simulink model "fivezonevav"  (R2020a)
settings: Solver=FixedStepAuto  StartTime=0  StopTime=2*24*3600  FixedStep=0.1  RelTol=1e-3
PostLoadFcn:
  | if any(exist('dsrtsu_mdlpostloadfcn', 'file') ~= 0), dsrtsu_mdlpostloadfcn('Execute', bdroot); end
InitFcn:
  | , if any(exist('rtifpga_mdlclblib', 'file') ~= 0), rtifpga_mdlclblib('Init', bdroot); end,
  | , if any(exist('dsmpb_private', 'file') ~= 0), dsmpb_private('dsmpb_mdlclblib', 'Init', bdroot); end,
undefined symbols (not defined in the file): dspaceexample_f_dy9753g2x2M
PreSaveFcn:
  | , if any(exist('dsmpb_private', 'file') ~= 0), dsmpb_private('dsmpb_mdlclblib', 'PreSave', bdroot); end,
CloseFcn:
  | , if any(exist('dsmpb_private', 'file') ~= 0), dsmpb_private('dsmpb_mdlclblib', 'Close', bdroot); end,
settings Model: RTICANMMDATA=struct('GeneralSetupData',struct('modelroot','D:\github\dspace-modelica-example\simulink\fivezone','generalsettings',struct('filesettings',struct('destfolder',struct('Name','RTICANMM_FILES','Check',1),'buildfolder',struct('Name','.','Check',1),'AbsDestfolder',struct('Name','D:\github\dspace-modelica-example\simulink\fivezone\RTICANMM_FILES'),'AbsBuildfolder',struct('Name','D:\github\dspace-modelica-example\simulink\fivezone'))),'options',struct('addpaths',1,'rmpaths',1,'addtrcexclusion',true,'cannavigator',struct('checkmonitoring',0),'show_usrtrc',0,'use_usrtrc',0),'advanced',struct('options',ones(1,100)),'MPSetup',{{}},'RTI',struct('Type','DSRT','Ver','4.3','Date','02-May-2020'),'modelname','fivezonevav','block','fivezonevav'))  DSRTSU_INTERNAL_RTIFPGA=160  DSMPB_ID_DATA={'100',struct('BlockId','6dd11bb4-ebec-4f08-8ba6-7ddbcbec7d3b','SignalIds',{{'2fb2bb90-4ec6-48ad-8f81-f1d196760c71'}}),'101',struct('BlockId','2ef807c6-571a-44f3-9a64-946af00fb830','SignalIds',{{'b929fcdd-48af-480b-af6b-b2c3ef490cf9'}}),'102',struct('BlockId','fcb8ffc9-48d0-43e3-97e6-63db34e8a87a','SignalIds',{{'7405cf0b-34b8-4d18-b681-bf257a32f1fc'}}),'103',struct('BlockId','44e3c1f1-df5a-4dd4-b5d4-1957fbd80a33','SignalIds',{{'7449a4d7-6efa-496e-ad1d-0eb127210326'}}),'104',struct('BlockId','d3fc6cbc-e5ea-45da-a1ff-e6d33e572c72','SignalIds',{{'ae88789f-7deb-4ded-bc5a-6d8a92166d0d'}}),'199',struct('BlockId','9376efae-c5ba-4aee-a189-875ca35da0c2','SignalIds',{{'13f0521d-e993-4fe3-8f8d-d5fdd3bf7eee'}}),'200',struct('BlockId','0e030ddc-3f5d-48b0-903c-79a8b3e79f79','SignalIds',{{'2dba2b15-4113-4beb-a147-18d9996277b5'}}),'595',struct('BlockId','6d740513-e981-40db-8ef0-eca4584907ef','SignalIds',{{'62a967d6-85c8-41d1-b978-878b95749907'}}),'596',struct('BlockId','7410bf17-4b2d-4b06-b0db-1a52506678f0','SignalIds',{{'4b878102-3f7f-4063-a0ae-65f2f571217e'}}),'97',struct('BlockId','c439f065-e928-4c50-b5e3-14eb295499a2','SignalIds',{{'8fe5f31b-da93-4239-8dda-b4cd2b1e3d5b'}}),'98',struct('BlockId','8b35e11d-29bf-41ba-bcb3-e0861426f11f','SignalIds',{{'ce953cd3-6947-465f-be2f-d959c5a96f49'}}),'99',struct('BlockId','4007e34d-3596-41e8-9571-21578a657730','SignalIds',{{'6190f487-0612-4ce8-bb29-664a6f7d7b4d'}})}  Creator=yangyang.fu  LastModifiedBy=yangyang.fu
settings OptimizationCC: BlockReduction=off  ConditionallyExecuteInputs=off  OptimizeBlockIOStorage=off  BufferReuse=off
settings DebuggingCC: TasksWithSamePriorityMsg=none
settings HardwareCC: ProdBitPerPointer=32  ProdBitPerSizeT=32  ProdBitPerPtrDiffT=32  ProdLargestAtomicInteger=Integer  ProdWordSize=32  ProdLongLongMode=on  ProdHWDeviceType=Custom Processor->Custom
settings ModelReferenceCC: EnableParallelModelReferenceBuilds=on
settings SFSimCC: MATLABDynamicMemAlloc=off
settings RTWCC: Description=dSPACE Run-Time Target (for VEOS on Windows and ConfigurationDesk)  SystemTargetFile=dsrt.tlc  GenCodeOnly=on  MakeCommand=make_dsrt  TemplateMakefile=dsrt_default_tmf  RTWVerbose=off  CustomInclude="\"C:\\Program Files\\Dymola 2021\\Source\""
settings STFCustomTargetCC: TargetLangStandard=C99 (ISO)  ParMdlRefBuildCompliant=on  SystemTargetFile=dsrt.tlc
settings GRTTargetCC: CompOptLevelCompliant=off  ConcurrentExecutionCompliant=off  CombineOutputUpdateFcns=off  MatFileLogging=off  CPPClassGenCompliant=off  UseToolchainInfoCompliant=off

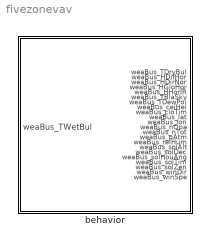
== system fivezonevav ==
  behavior : Subsystem  Tag=03-Feb-2022 00:05:26#975  LoadFcn=if exist('newDymolaGui') newDymolaGui('fivezonevav/behavior','PostLoadNew'); else error('Dymola not installed. Must install at least the file newDymolaGui.p'); end;
      mask help:
      | Dymola block.
      | A dymola block allows acausal physical modeling.
      | See Dymola manual for usage.
      settings: CopyFcn=newDymolaGui('03-Feb-2022 00:05:26#975','Copy');  DeleteFcn=if exist('newDymolaGui') newDymolaGui('fivezonevav/behavior','Delete'); end;  NameChangeFcn=newDymolaGui('03-Feb-2022 00:05:26#975','Copy');  OpenFcn=newDymolaGui('fivezonevav/behavior','Init');
      mask Display: image(reshape([1;1;1;1;1;1;1;1;1;1;1;1;1;1;1;1;1;1;1;1;1;1;0;0;0;0;0;0;0;0;0;0;1;1;1;1;1;1;1;1;0;1;1;1;1;1;1;1;1;0;1;1;1;1;1;0;0;0;0;0;0;0;1;1;0;0;0;0;0;0;0;1;1;0;0;0;0;0;0;0;1;1;0;0;0;0;0;0;0;1;1;0;0;0;0;0;0;0;1;1;0;0;0;0;0;0;0;1;1;0;0;0;0;0;0;0;1;1;0;0;0;0;0;0;0;1;1;0;0;0;0;0;0;0;1;1;0;0;0;0;0;0;0;1;1;0;0;0;0;0;0;0;1;1;0;0;0;0;0;0;0;1;1;0;0;0;0;0;0;0;1;1;0;0;0;0;0;0;0;1;1;0;0;0;0;0;0;0;1;1;0;0;0;0;0;0;0;1;1;0;0;0;0;0;0;0;1;1;0;0;0;0;0;0;0;1;1;0;0;0;0;0;0;0;1;1;0;0;0;0;0;0;0;1;1;0;0;0;0;0;0;0;1;1;0;0;0;0;0;0;0;1;1;0;0;0;0;0;0;0;1;1;0;0;0;0;0;0;0;1;1;1;1;1;0;1;1;1;1;1;1;1;1;0;1;1;1;1;1;1;1;1;0;0;0;0;0;0;0;0;0;0;1;1;1;1;1;1;1;1;1;1;1;1;1;1;1;1;1;1;1;1;1;1;1;1;1;1;1;1;1;1;1;1;1;1;1;1;1;1;1;1;1;1;1;1;0;0;0;0;0;0;0;0;0;0;1;1;1;1;1;1;1;1;0;1;1;1;1;1;1;1;1;0;1;1;1;1;1;0;0;0;0;0;0;0;1;1;0;0;0;0;0;0;0;1;1;0;0;0;0;0;0;0;1;1;0;0;0;0;0;0;0;1;1;0;0;0;0;0;0;0;1;1;0;0;0;0;0;0;0;1;1;0;0;0;0;0;0;0;1;1;0;0;0;0;0;0;0;1;1;0;0;0;0;0;0;0;1;1;0;0;0;0;0;0;0;1;1;0;0;0;0;0;0;0;1;1;0;0;0;0;0;0;0;1;1;0;0;0;0;0;0;0;1;1;0;0;0;0;0;0;0;1;1;0;0;0;0;0;0;0;1;1;0;0;0;0;0;0;0;1;1;0;0;0;0;0;0;0;1;1;0;0;0;0;0;0;0;1;1;0;0;0;0;0;0;0;1;1;0;0;0;0;0;0;0;1;1;0;0;0;0;0;0;0;1;1;0;0;0;0;0;0;0;1;1;0;0;0;0;0;0;0;1;1;0;0;0;0;0;0;0;1;1;1;1;1;0;1;1;1;1;1;1;1;1;0;1;1;1;1;1;1;1;1;0;0;0;0;0;0;0;0;0;0;1;1;1;1;1;1;1;1;1;1;1;1;1;1;1;1;1;1;1;1;1;1;1;1;1;1;1;1;1;1;1;1;1;1;1;1;1;1;1;1;1;1;1;1;0;0;0;0;0;0;0;0;0;0;1;1;1;1;1;1;1;1;0;1;1;1;1;1;1;1;1;0;1;1;1;1;1;0;0;0;0;0;0;0;1;1;0;0;0;0;0;0;0;1;1;0;1;1;1;1;1;0;1;1;0;1;1;1;1;1;0;1;1;0;1;1;1;1;1;0;1;1;0;1;1;1;1;1;0;1;1;0;1;1;1;1;1;0;1;1;0;1;1;1;1;1;0;1;1;0;1;1;1;1;1;0;1;1;0;1;1;1;1;1;0;1;1;0;1;1;1;1;1;0;1;1;0;1;1;1;1;1;0;1;1;0;1;1;1;1;1;0;1;1;0;1;1;1;1;1;0;1;1;0;1;1;1;1;1;0;1;1;0;1;1;1;1;1;0;1;1;0;1;1;1;1;1;0;1;1;0;1;1;1;1;1;0;1;1;0;1;1;1;1;1;0;1;1;0;1;1;1;1;1;0;1;1;0;1;1;1;1;1;0;1;1;0;1;1;1;1;1;0;1;1;0;0;0;0;0;0;0;1;1;0;0;0;0;0;0;0;1;1;1;1;1;0;1;1;1;1;1;1;1;1;0;1;1;1;1;1;1;1;1;0;0;0;0;0;0;0;0;0;0;1;1;1;1;1;1;1;1;1;1;1;1;1;1;1;1;1;1;1;1;1;1],18,18,3),[.2,.2,.6,.6])

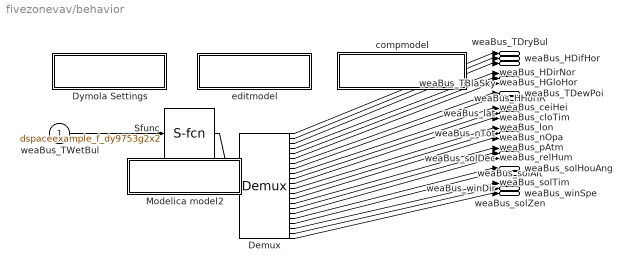
== system fivezonevav/behavior ==
  weaBus_TWetBul : Inport
  Demux : Demux  Outputs=[1;1;1;1;1;1;1;1;1;1;1;1;1;1;1;1;1;1;1;1;1;1]
  Dymola Settings : Subsystem  mask{ModelName=dSpaceExample.FiveZones.BaselineSystem, MoFileName=D:/github/dspace-modelica-example/dSpaceExample/FiveZones/BaselineSystem.mo, dSpace=, BusConnector=[], ResultFile=[], ResultFileOnline=[], ResultDt=[], Libs=:, bigobj=[], ImportFolder=[], guimode=[], ModelName2=[], forRuntime=[], MEXLoad=[], omitDescription=[], ResultName=dspaceexample_f_dy9753g2x2}
      mask prompts: ModelName "Name of Dymola model"; MoFileName "File Name (including .mo)"; ResultFile "Create Result"; ResultFileOnline "Load result"; ResultDt "Result min dt"; Libs "Used Libraries"; bigobj "Compiler flag /bigobj"; ImportFolder "Import folder"; guimode "GUI mode flag"; ModelName2 "Model name for import mode"; forRuntime "Runtime export"; MEXLoad "Compiled S-function"; omitDescription "Omit description strings"; ResultName "Name of result file"
      mask Display: disp('Dymola Settings');
  Modelica model2 : Subsystem
      mask Display: disp('Change parameters');
  Sfunc : S-Function  Tag=9753g2x2  FunctionName=dspaceexample_f_dy9753g2x2  Parameters=[dspaceexample_f_dy9753g2x2M.pV],[dspaceexample_f_dy9753g2x2M.x0V]  PortCounts=[1;1]  SFunctionDeploymentMode=off  EnableBusSupport=off
      mask Display: image(imread('Dymola.bmp'))
  compmodel : Subsystem
      settings: OpenFcn=compileModelica('fivezonevav/behavior');
      mask Display: disp('Compile Modelica model');
  editmodel : Subsystem
      settings: OpenFcn=editModelica('fivezonevav/behavior');
      mask Display: disp('Edit Modelica model');
  weaBus_TDryBul : Outport
  weaBus_HDifHor : Outport  Port=2
  weaBus_HDirNor : Outport  Port=3
  weaBus_HGloHor : Outport  Port=4
  weaBus_HHorIR : Outport  Port=5
  weaBus_TBlaSky : Outport  Port=6
  weaBus_TDewPoi : Outport  Port=7
  weaBus_ceiHei : Outport  Port=8
  weaBus_cloTim : Outport  Port=9
  weaBus_lat : Outport  Port=10
  weaBus_lon : Outport  Port=11
  weaBus_nOpa : Outport  Port=12
  weaBus_nTot : Outport  Port=13
  weaBus_pAtm : Outport  Port=14
  weaBus_relHum : Outport  Port=15
  weaBus_solAlt : Outport  Port=16
  weaBus_solDec : Outport  Port=17
  weaBus_solHouAng : Outport  Port=18
  weaBus_solTim : Outport  Port=19
  weaBus_solZen : Outport  Port=20
  weaBus_winDir : Outport  Port=21
  weaBus_winSpe : Outport  Port=22
  wires:
  Sfunc/1 -> Demux/1
  Demux/1 -> weaBus_TDryBul/1
  Demux/2 -> weaBus_HDifHor/1
  Demux/3 -> weaBus_HDirNor/1
  Demux/4 -> weaBus_HGloHor/1
  Demux/5 -> weaBus_HHorIR/1
  Demux/6 -> weaBus_TBlaSky/1
  Demux/7 -> weaBus_TDewPoi/1
  Demux/8 -> weaBus_ceiHei/1
  Demux/9 -> weaBus_cloTim/1
  Demux/10 -> weaBus_lat/1
  Demux/11 -> weaBus_lon/1
  Demux/12 -> weaBus_nOpa/1
  Demux/13 -> weaBus_nTot/1
  Demux/14 -> weaBus_pAtm/1
  Demux/15 -> weaBus_relHum/1
  Demux/16 -> weaBus_solAlt/1
  Demux/17 -> weaBus_solDec/1
  Demux/18 -> weaBus_solHouAng/1
  Demux/19 -> weaBus_solTim/1
  Demux/20 -> weaBus_solZen/1
  Demux/21 -> weaBus_winDir/1
  Demux/22 -> weaBus_winSpe/1
  weaBus_TWetBul/1 -> Sfunc/1

== system fivezonevav/behavior/Dymola Settings ==

== system fivezonevav/behavior/Modelica model2 ==

== system fivezonevav/behavior/compmodel ==

== system fivezonevav/behavior/editmodel ==
